simulink model "f14_digital"  (Simulink 7.6)
settings: Solver=ode45  SolverMode=SingleTasking  StartTime=0.0  StopTime=60  FixedStep=.01  RelTol=1e-4  AbsTol=1e-6
PreLoadFcn:
  | load f14_digital_data.mat
values from neighbouring files (symbols this model uses):
  a = 2.5348    [f14_digital_data.mat]    (also in f14dat_digital.m; sanim.m = size(vert); sanim3dof.m = size(vert))
  b = 64.13    [f14_digital_data.mat]    (also in f14dat_digital.m)
  deltat = pinput(23)    [aero_extkalman.m]    (also in aero_radplot.m = 1; f14_digital_data.mat = 0.1; f14dat_digital.m = 0.1)
  deltat1 = 0.01    [f14_digital_data.mat]    (also in f14dat_digital.m)
  fden = [1 188.495559215 17765.287922 837169.470368]    [f14_digital_data.mat]    (also in f14dat_digital.m = [ 1, 1.884955592153875e+02, 1.776528792196083e+04, 8.3716947)
  fnum = [0 0 0 837169.470368]    [f14_digital_data.mat]    (also in f14dat_digital.m = [ 0, 0, 0, 8.371694703680943e+05 ])
  g = 9.81    [aero_guid_dat.m]    (also in f14_digital_data.mat = 32.2; f14dat_digital.m = 32.2)
  Ka = 0.677    [f14_digital_data.mat]    (also in f14dat_digital.m)
  Kf = -1.746    [f14_digital_data.mat]    (also in f14dat_digital.m)
  Ki = -3.864    [f14_digital_data.mat]    (also in f14dat_digital.m)
  Kq = 0.8156    [f14_digital_data.mat]    (also in f14dat_digital.m)
  Md = -6.8847    [f14_digital_data.mat]    (also in f14dat_digital.m)
  Mq = -0.6571    [f14_digital_data.mat]    (also in f14dat_digital.m)
  Mw = -0.00592    [f14_digital_data.mat]    (also in f14dat_digital.m)
  Swg = 3    [f14_digital_data.mat]    (also in f14dat_digital.m)
  Tal = 0.3959    [f14_digital_data.mat]    (also in f14dat_digital.m)
  Ts = 0.1    [f14_digital_data.mat]    (also in f14dat_digital.m)
  Uo = 689.4    [f14_digital_data.mat]    (also in f14dat_digital.m)
  Vto = 690.4    [f14_digital_data.mat]    (also in f14dat_digital.m)
  W1 = 2.971    [f14_digital_data.mat]    (also in f14dat_digital.m)
  W2 = 4.144    [f14_digital_data.mat]    (also in f14dat_digital.m)
  Zd = -63.9979    [f14_digital_data.mat]    (also in f14dat_digital.m)
  Zw = -0.6385    [f14_digital_data.mat]    (also in f14dat_digital.m)
undefined symbols (not defined in the file or in its folder): DiscIntNeverNeededParam
libraries: simulink x5, f14actuator x1, cstblocks x1
Description:
  | High angle of attack mode for a digital flight control system
settings Model: Creator=The MathWorks Inc.  ExtModeTrigMode=oneshot  ExtModeArmWhenConnect=off  ExtModeAutoUpdateStatusClock=off
settings DataIOCC: ExternalInput=[]  InitialState=[]  LimitDataPoints=off  SaveOutput=off  SaveTime=off  SignalLoggingName=logsOut
settings OptimizationCC: BlockReduction=off  BooleanDataType=off  InlineInvariantSignals=on  InitFltsAndDblsToZero=on
settings DebuggingCC: SaveWithParameterizedLinksMsg=none  CheckExecutionContextPreStartOutputMsg=on  CheckExecutionContextRuntimeOutputMsg=on  SignalResolutionControl=TryResolveAllWithWarning  SolverPrmCheckMsg=none  MultiTaskDSMMsg=warning  MultiTaskCondExecSysMsg=none  SigSpecEnsureSampleTimeMsg=none  IntegerOverflowMsg=none
settings SFSimCC: SimParseCustomCode=off
settings RTWCC: GenCodeOnly=on  TemplateMakefile=grt_vc.tmf  IncludeERTFirstTime=on
settings CodeAppCC: CustomSymbolStrFcn=$F$N$M
settings GRTTargetCC: TargetFcnLib=ansi_tfl_tmw.mat

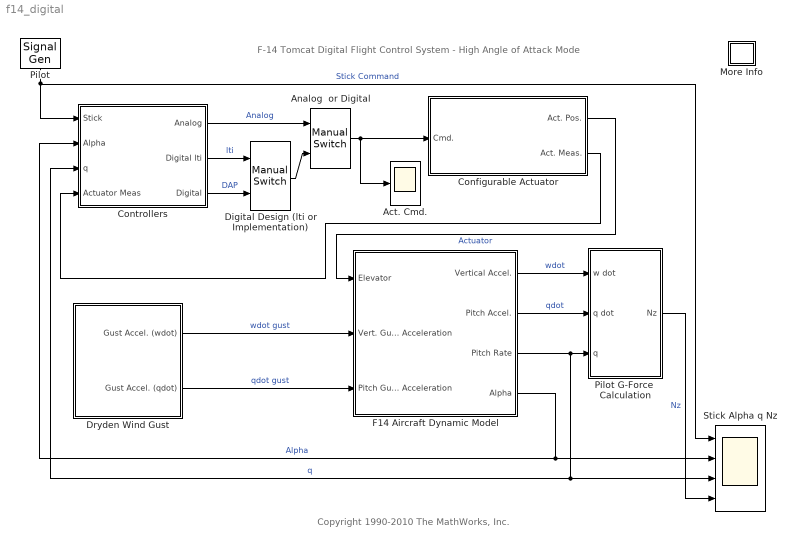
== system f14_digital ==
  note: Copyright 1990-2010 The MathWorks, Inc.
  note: F-14 Tomcat Digital Flight Control System - High Angle of Attack Mode
  Act. Cmd. : Scope
      settings: TickLabels=on  TimeRange=15  YMin=-2.5  YMax=2.5  DataFormat=Array
  Analog  or Digital : simulink/Signal Routing/Manual Switch  SystemSampleTime=-1  sw=1  action=0  varsize=off
  Configurable Actuator : Subsystem  BlockChoice=Linear Actuator Subsystem
      settings: MemberBlocks=Linear Actuator Subsystem,Non-Linear Actuator Subsystem
      settings: TemplateBlock=|
      | f14actuator/Configurable
      | Actuator
  Controllers : Subsystem
      mask Display: image(evalin('base','contrgb'))
  Digital Design (lti or Implementation) : simulink/Signal Routing/Manual Switch  SystemSampleTime=-1  sw=0  action=0  varsize=off
  Dryden Wind Gust : Subsystem
      mask Display: image(evalin('base','weatherrgb'))
  F14 Aircraft Dynamic Model : Subsystem
      mask Display: image(evalin('base','rgb'))
  More Info : Subsystem
      settings: OpenFcn=showdemo(bdroot(gcb))
      mask Display: disp('?')
  Pilot : SignalGenerator  WaveForm=square  Frequency=.1
  Pilot G-Force  Calculation : Subsystem
  Stick Alpha q Nz : Scope  NumInputPorts=4
      settings: TickLabels=on  TimeRange=15  YMin=-1~-1.5~-3~-15  YMax=1~1.5~3~15  DataFormat=Array
  wires:
  Controllers/3(Digital) -> Digital Design (lti or Implementation)/2  "DAP"
  Controllers/2(Digital lti) -> Digital Design (lti or Implementation)/1  "lti"
  Digital Design (lti or Implementation)/1 -> Analog  or Digital/2
  Configurable Actuator/1(Act. Pos.) -> F14 Aircraft Dynamic Model/1(Elevator)  "Actuator"
  Controllers/1(Analog) -> Analog  or Digital/1  "Analog"
  F14 Aircraft Dynamic Model/1(Vertical Accel.) -> Pilot G-Force  Calculation/1(w dot)  "wdot"
  F14 Aircraft Dynamic Model/2(Pitch Accel.) -> Pilot G-Force  Calculation/2(q dot)  "qdot"
  Pilot/1 -> Stick Alpha q Nz/1, Controllers/1(Stick)  "Stick Command"
  F14 Aircraft Dynamic Model/4(Alpha) -> Stick Alpha q Nz/2, Controllers/2(Alpha)  "Alpha"
  Configurable Actuator/2(Act. Meas.) -> Controllers/4(Actuator Meas)
  Dryden Wind Gust/2(Gust Accel. (qdot)) -> F14 Aircraft Dynamic Model/3(Pitch Gust Acceleration)  "qdot gust"
  Dryden Wind Gust/1(Gust Accel. (wdot)) -> F14 Aircraft Dynamic Model/2(Vert. Gust Acceleration)  "wdot gust"
  F14 Aircraft Dynamic Model/3(Pitch Rate) -> Pilot G-Force  Calculation/3(q), Stick Alpha q Nz/3, Controllers/3(q)  "q"
  Pilot G-Force  Calculation/1(Nz) -> Stick Alpha q Nz/4  "Nz"
  Analog  or Digital/1 -> Configurable Actuator/1(Cmd.), Act. Cmd./1

== system f14_digital/Configurable Actuator ==
  Cmd. : Inport
  Linear Actuator Subsystem : f14actuator/Linear Actuator Subsystem  SystemSampleTime=-1
  Act. Pos. : Outport
  Act. Meas. : Outport  Port=2
  wires:
  Cmd./1 -> Linear Actuator Subsystem/1
  Linear Actuator Subsystem/1 -> Act. Pos./1
  Linear Actuator Subsystem/2 -> Act. Meas./1

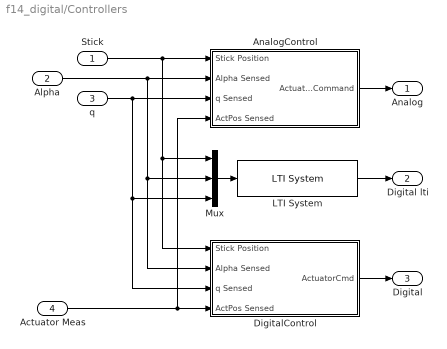
== system f14_digital/Controllers ==
  Stick : Inport
  Alpha : Inport  Port=2
  q : Inport  Port=3
  Actuator Meas : Inport  Port=4
  AnalogControl : Subsystem
  DigitalControl : Subsystem
  LTI System : cstblocks/LTI System  sys=discap  IC=[0]
  Mux : Mux  Inputs=3
  Analog : Outport
  Digital lti : Outport  Port=2
  Digital : Outport  Port=3
  wires:
  Stick/1 -> AnalogControl/1(Stick Position), DigitalControl/1(Stick Position), Mux/1
  Actuator Meas/1 -> DigitalControl/4(ActPos Sensed), AnalogControl/4(ActPos Sensed)
  LTI System/1 -> Digital lti/1
  DigitalControl/1(ActuatorCmd) -> Digital/1
  AnalogControl/1(Actuator Command) -> Analog/1
  Mux/1 -> LTI System/1
  Alpha/1 -> AnalogControl/2(Alpha Sensed), DigitalControl/2(Alpha Sensed), Mux/2
  q/1 -> AnalogControl/3(q Sensed), DigitalControl/3(q Sensed), Mux/3

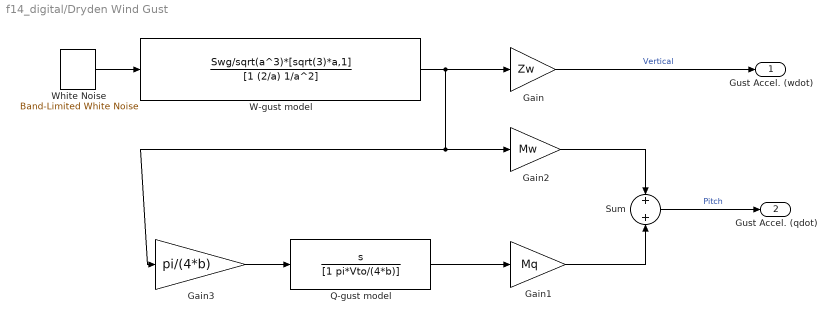
== system f14_digital/Dryden Wind Gust ==
  Gain : Gain  Gain=Zw  SaturateOnIntegerOverflow=on  OutDataTypeStr=Inherit: Same as input  ParamDataTypeStr=Inherit: Same as input
  Gain1 : Gain  Gain=Mq  SaturateOnIntegerOverflow=on  OutDataTypeStr=Inherit: Same as input  ParamDataTypeStr=Inherit: Same as input
  Gain2 : Gain  Gain=Mw  SaturateOnIntegerOverflow=on  OutDataTypeStr=Inherit: Same as input  ParamDataTypeStr=Inherit: Same as input
  Gain3 : Gain  Gain=pi/(4*b)  SaturateOnIntegerOverflow=on  OutDataTypeStr=Inherit: Same as input  ParamDataTypeStr=Inherit: Same as input
  Q-gust model : TransferFcn  Numerator=[1 0]  Denominator=[1 pi*Vto/(4*b)]
  Sum : Sum  SaturateOnIntegerOverflow=on  InputSameDT=on  OutDataTypeStr=Inherit: Same as first input
  W-gust model : TransferFcn  Numerator=Swg/sqrt(a^3)*[sqrt(3)*a,1]  Denominator=[1 (2/a) 1/a^2]
  White Noise : simulink/Sources/Band-Limited White Noise  Cov=10  Ts=0.01  seed=23341
  Gust Accel. (wdot) : Outport
  Gust Accel. (qdot) : Outport  Port=2
  wires:
  Gain/1 -> Gust Accel. (wdot)/1  "Vertical"
  White Noise/1 -> W-gust model/1
  Gain3/1 -> Q-gust model/1
  Sum/1 -> Gust Accel. (qdot)/1  "Pitch"
  Gain2/1 -> Sum/1
  Gain1/1 -> Sum/2
  Q-gust model/1 -> Gain1/1
  W-gust model/1 -> Gain/1, Gain2/1, Gain3/1

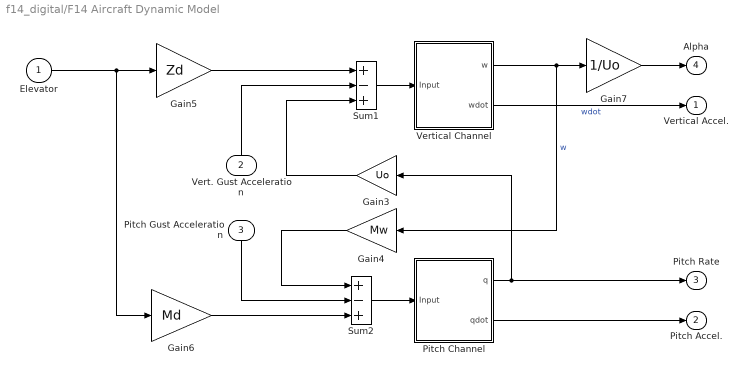
== system f14_digital/F14 Aircraft Dynamic Model ==
  Elevator : Inport
  Vert. Gust Acceleration : Inport  Port=2
  Pitch Gust Acceleration : Inport  Port=3
  Gain3 : Gain  Gain=Uo  SaturateOnIntegerOverflow=on  OutDataTypeStr=Inherit: Same as input  ParamDataTypeStr=Inherit: Same as input
  Gain4 : Gain  Gain=Mw  SaturateOnIntegerOverflow=on  OutDataTypeStr=Inherit: Same as input  ParamDataTypeStr=Inherit: Same as input
  Gain5 : Gain  Gain=Zd  SaturateOnIntegerOverflow=on  OutDataTypeStr=Inherit: Same as input  ParamDataTypeStr=Inherit: Same as input
  Gain6 : Gain  Gain=Md  SaturateOnIntegerOverflow=on  OutDataTypeStr=Inherit: Same as input  ParamDataTypeStr=Inherit: Same as input
  Gain7 : Gain  Gain=1/Uo  SaturateOnIntegerOverflow=on  OutDataTypeStr=Inherit: Same as input  ParamDataTypeStr=Inherit: Same as input
  Pitch Channel : Subsystem
  Sum1 : Sum  Inputs=+-+  SaturateOnIntegerOverflow=on  InputSameDT=on  OutDataTypeStr=Inherit: Same as first input
  Sum2 : Sum  Inputs=+-+  SaturateOnIntegerOverflow=on  InputSameDT=on  OutDataTypeStr=Inherit: Same as first input
  Vertical Channel : Subsystem
  Vertical Accel. : Outport
  Pitch Accel. : Outport  Port=2
  Pitch Rate : Outport  Port=3
  Alpha : Outport  Port=4
  wires:
  Pitch Channel/2(qdot) -> Pitch Accel./1
  Pitch Channel/1(q) -> Pitch Rate/1, Gain3/1
  Vertical Channel/2(wdot) -> Vertical Accel./1  "wdot"
  Vertical Channel/1(w) -> Gain4/1, Gain7/1  "w"
  Sum1/1 -> Vertical Channel/1(Input)
  Gain6/1 -> Sum2/3
  Gain5/1 -> Sum1/1
  Pitch Gust Acceleration/1 -> Sum2/2
  Sum2/1 -> Pitch Channel/1(Input)
  Vert. Gust Acceleration/1 -> Sum1/2
  Elevator/1 -> Gain5/1, Gain6/1
  Gain7/1 -> Alpha/1
  Gain3/1 -> Sum1/3
  Gain4/1 -> Sum2/1

== system f14_digital/More Info ==

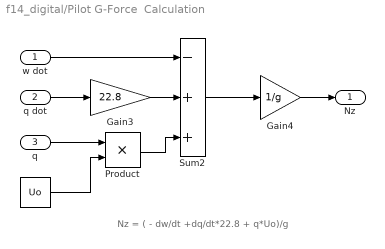
== system f14_digital/Pilot G-Force  Calculation ==
  note: Nz = ( - dw/dt +dq/dt*22.8 + q*Uo)/g
  w dot : Inport
  q dot : Inport  Port=2
  q : Inport  Port=3
  " " : Constant  Value=Uo
  Gain3 : Gain  Gain=22.8  SaturateOnIntegerOverflow=on  OutDataTypeStr=Inherit: Same as input  ParamDataTypeStr=Inherit: Same as input
  Gain4 : Gain  Gain=1/g  SaturateOnIntegerOverflow=on  OutDataTypeStr=Inherit: Same as input  ParamDataTypeStr=Inherit: Same as input
  Product : Product  SaturateOnIntegerOverflow=on  RndMeth=Zero  InputSameDT=on  OutDataTypeStr=Inherit: Same as first input
  Sum2 : Sum  Inputs=-++  SaturateOnIntegerOverflow=on  InputSameDT=on  OutDataTypeStr=Inherit: Same as first input
  Nz : Outport
  wires:
  Sum2/1 -> Gain4/1
  w dot/1 -> Sum2/1
  Gain4/1 -> Nz/1
  q dot/1 -> Gain3/1
  Gain3/1 -> Sum2/2
  Product/1 -> Sum2/3
  q/1 -> Product/1
  " "/1 -> Product/2

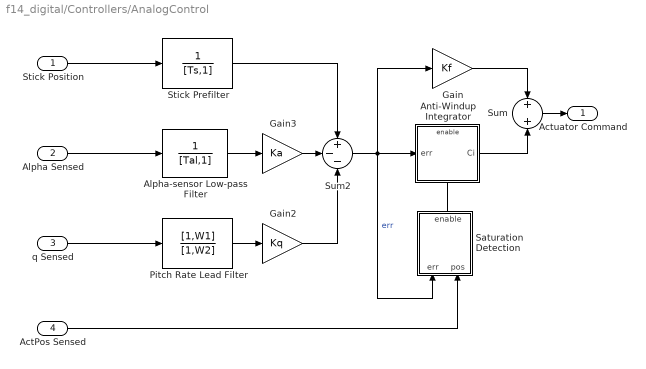
== system f14_digital/Controllers/AnalogControl ==
  Stick Position : Inport
  Alpha Sensed : Inport  Port=2
  q Sensed : Inport  Port=3
  ActPos Sensed : Inport  Port=4
  Alpha-sensor Low-pass Filter : TransferFcn  Denominator=[Tal,1]
  Anti-Windup Integrator : Subsystem  TreatAsAtomicUnit=on
      settings: RTWSystemCode=Inline
  Gain : Gain  Gain=Kf  SaturateOnIntegerOverflow=on  OutDataTypeStr=Inherit: Same as input  ParamDataTypeStr=Inherit: Same as input
  Gain2 : Gain  Gain=Kq  SaturateOnIntegerOverflow=on  OutDataTypeStr=Inherit: Same as input  ParamDataTypeStr=Inherit: Same as input
  Gain3 : Gain  Gain=Ka  SaturateOnIntegerOverflow=on  OutDataTypeStr=Inherit: Same as input  ParamDataTypeStr=Inherit: Same as input
  Pitch Rate Lead Filter : TransferFcn  Numerator=[1,W1]  Denominator=[1,W2]
  Saturation Detection : Subsystem
  Stick Prefilter : TransferFcn  Denominator=[Ts,1]
  Sum : Sum  Inputs=2  SaturateOnIntegerOverflow=on  InputSameDT=on  OutDataTypeStr=Inherit: Same as first input
  Sum2 : Sum  Inputs=+--  SaturateOnIntegerOverflow=on  InputSameDT=on  OutDataTypeStr=Inherit: Same as first input
  Actuator Command : Outport
  wires:
  Sum2/1 -> Gain/1, Anti-Windup Integrator/1(err), Saturation Detection/1(err)  "err"
  Anti-Windup Integrator/1(Ci) -> Sum/2
  Sum/1 -> Actuator Command/1
  Stick Position/1 -> Stick Prefilter/1
  Alpha-sensor Low-pass Filter/1 -> Gain3/1
  Gain2/1 -> Sum2/3
  Stick Prefilter/1 -> Sum2/1
  Pitch Rate Lead Filter/1 -> Gain2/1
  Gain3/1 -> Sum2/2
  Gain/1 -> Sum/1
  Alpha Sensed/1 -> Alpha-sensor Low-pass Filter/1
  q Sensed/1 -> Pitch Rate Lead Filter/1
  ActPos Sensed/1 -> Saturation Detection/2(pos)
  Saturation Detection/1(enable) -> Anti-Windup Integrator/Enable

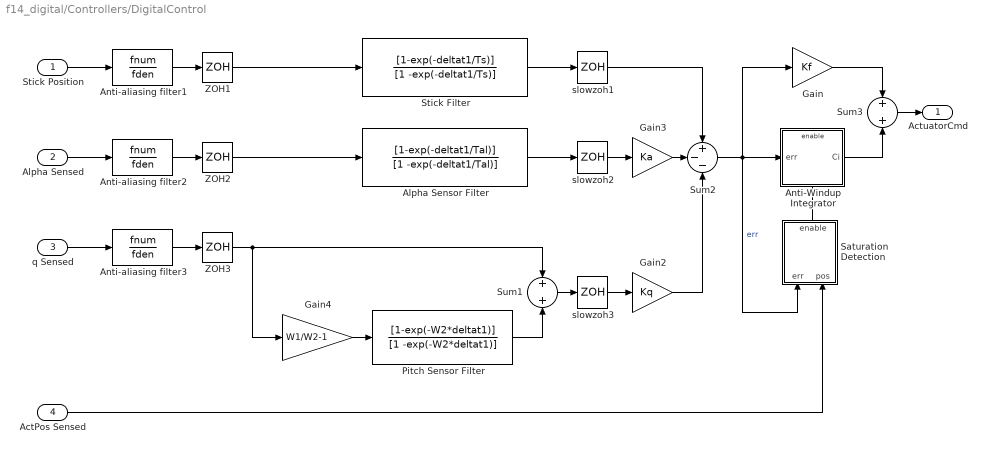
== system f14_digital/Controllers/DigitalControl ==
  Stick Position : Inport
  Alpha Sensed : Inport  Port=2
  q Sensed : Inport  Port=3
  ActPos Sensed : Inport  Port=4
  Alpha Sensor Filter : DiscreteTransferFcn  Numerator=[1-exp(-deltat1/Tal)]  Denominator=[1 -exp(-deltat1/Tal)]  SampleTime=deltat1
  Anti-Windup Integrator : Subsystem  TreatAsAtomicUnit=on
      settings: RTWSystemCode=Inline
  Anti-aliasing filter1 : TransferFcn  Numerator=fnum  Denominator=fden
      settings: AttributesFormatString=%<Description>
  Anti-aliasing filter2 : TransferFcn  Numerator=fnum  Denominator=fden
      settings: AttributesFormatString=%<Description>
  Anti-aliasing filter3 : TransferFcn  Numerator=fnum  Denominator=fden
      settings: AttributesFormatString=%<Description>
  Gain : Gain  Gain=Kf  SaturateOnIntegerOverflow=on  OutDataTypeStr=Inherit: Same as input  ParamDataTypeStr=Inherit: Same as input
  Gain2 : Gain  Gain=Kq  SaturateOnIntegerOverflow=on  OutDataTypeStr=Inherit: Same as input  ParamDataTypeStr=Inherit: Same as input
  Gain3 : Gain  Gain=Ka  SaturateOnIntegerOverflow=on  OutDataTypeStr=Inherit: Same as input  ParamDataTypeStr=Inherit: Same as input
  Gain4 : Gain  Gain=W1/W2-1  SaturateOnIntegerOverflow=on  OutDataTypeStr=Inherit: Same as input  ParamDataTypeStr=Inherit: Same as input
  Pitch Sensor Filter : DiscreteTransferFcn  Numerator=[1-exp(-W2*deltat1)]  Denominator=[1 -exp(-W2*deltat1)]  SampleTime=deltat1
  Saturation Detection : Subsystem
  Stick Filter : DiscreteTransferFcn  Numerator=[1-exp(-deltat1/Ts)]  Denominator=[1 -exp(-deltat1/Ts)]  SampleTime=deltat1
  Sum1 : Sum  Inputs=2  SaturateOnIntegerOverflow=on  InputSameDT=on  OutDataTypeStr=Inherit: Same as first input
  Sum2 : Sum  Inputs=+--  SaturateOnIntegerOverflow=on  InputSameDT=on  OutDataTypeStr=Inherit: Same as first input
  Sum3 : Sum  Inputs=2  SaturateOnIntegerOverflow=on  InputSameDT=on  OutDataTypeStr=Inherit: Same as first input
  ZOH1 : ZeroOrderHold  SampleTime=deltat1
  ZOH2 : ZeroOrderHold  SampleTime=deltat1
  ZOH3 : ZeroOrderHold  SampleTime=deltat1
  slowzoh1 : ZeroOrderHold  SampleTime=deltat
  slowzoh2 : ZeroOrderHold  SampleTime=deltat
  slowzoh3 : ZeroOrderHold  SampleTime=deltat
  ActuatorCmd : Outport
  wires:
  Sum3/1 -> ActuatorCmd/1
  Sum2/1 -> Gain/1, Anti-Windup Integrator/1(err), Saturation Detection/1(err)  "err"
  Alpha Sensed/1 -> Anti-aliasing filter2/1
  Stick Filter/1 -> slowzoh1/1
  slowzoh1/1 -> Sum2/1
  Alpha Sensor Filter/1 -> slowzoh2/1
  slowzoh2/1 -> Gain3/1
  Gain3/1 -> Sum2/2
  Gain/1 -> Sum3/1
  Anti-Windup Integrator/1(Ci) -> Sum3/2
  Gain2/1 -> Sum2/3
  q Sensed/1 -> Anti-aliasing filter3/1
  Sum1/1 -> slowzoh3/1
  Pitch Sensor Filter/1 -> Sum1/2
  Gain4/1 -> Pitch Sensor Filter/1
  slowzoh3/1 -> Gain2/1
  Stick Position/1 -> Anti-aliasing filter1/1
  ZOH1/1 -> Stick Filter/1
  Anti-aliasing filter1/1 -> ZOH1/1
  Anti-aliasing filter2/1 -> ZOH2/1
  Anti-aliasing filter3/1 -> ZOH3/1
  ZOH2/1 -> Alpha Sensor Filter/1
  ZOH3/1 -> Sum1/1, Gain4/1
  Saturation Detection/1(enable) -> Anti-Windup Integrator/Enable
  ActPos Sensed/1 -> Saturation Detection/2(pos)

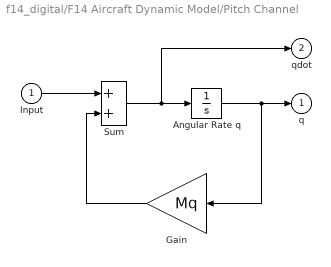
== system f14_digital/F14 Aircraft Dynamic Model/Pitch Channel ==
  Input : Inport
  "Angular Rate q " : Integrator
  Gain : Gain  Gain=Mq  SaturateOnIntegerOverflow=on  OutDataTypeStr=Inherit: Same as input  ParamDataTypeStr=Inherit: Same as input
  Sum : Sum  SaturateOnIntegerOverflow=on  InputSameDT=on  OutDataTypeStr=Inherit: Same as first input
  q : Outport
  qdot : Outport  Port=2
  wires:
  Input/1 -> Sum/1
  Gain/1 -> Sum/2
  "Angular Rate q "/1 -> q/1, Gain/1
  Sum/1 -> "Angular Rate q "/1, qdot/1

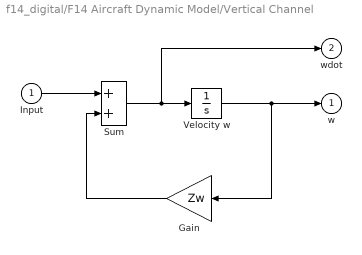
== system f14_digital/F14 Aircraft Dynamic Model/Vertical Channel ==
  Input : Inport
  Gain : Gain  Gain=Zw  SaturateOnIntegerOverflow=on  OutDataTypeStr=Inherit: Same as input  ParamDataTypeStr=Inherit: Same as input
  Sum : Sum  SaturateOnIntegerOverflow=on  InputSameDT=on  OutDataTypeStr=Inherit: Same as first input
  Velocity w : Integrator
  w : Outport
  wdot : Outport  Port=2
  wires:
  Sum/1 -> wdot/1, Velocity w/1
  Velocity w/1 -> Gain/1, w/1
  Gain/1 -> Sum/2
  Input/1 -> Sum/1

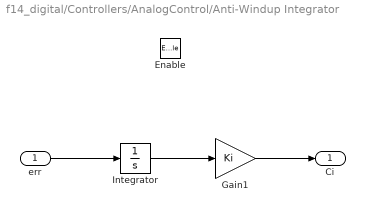
== system f14_digital/Controllers/AnalogControl/Anti-Windup Integrator ==
  err : Inport
  Enable : EnablePort
  Gain1 : Gain  Gain=Ki  SaturateOnIntegerOverflow=on  OutDataTypeStr=Inherit: Same as input  ParamDataTypeStr=Inherit: Same as input
  Integrator : Integrator
  Ci : Outport  InitialOutput=0
  wires:
  err/1 -> Integrator/1
  Integrator/1 -> Gain1/1
  Gain1/1 -> Ci/1

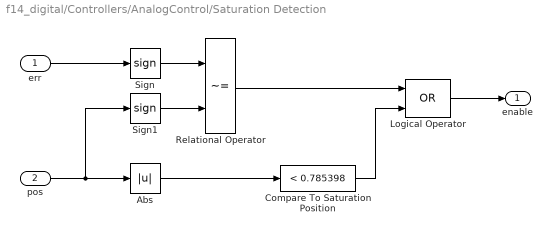
== system f14_digital/Controllers/AnalogControl/Saturation Detection ==
  err : Inport
  pos : Inport  Port=2
  Abs : Abs  ZeroCross=off
  Compare To Saturation Position : simulink/Logic and Bit Operations/Compare To Constant  relop=<  const=0.785398  LogicOutDataTypeMode=boolean  ZeroCross=off
  Logical Operator : Logic  Operator=OR  AllPortsSameDT=off  OutDataTypeStr=boolean
  Relational Operator : RelationalOperator  Operator=~=  OutDataTypeStr=boolean  ZeroCross=off
  Sign : Signum  ZeroCross=off
  Sign1 : Signum  ZeroCross=off
  enable : Outport
  wires:
  pos/1 -> Sign1/1, Abs/1
  Sign/1 -> Relational Operator/1
  Relational Operator/1 -> Logical Operator/1
  Compare To Saturation Position/1 -> Logical Operator/2
  Sign1/1 -> Relational Operator/2
  Abs/1 -> Compare To Saturation Position/1
  err/1 -> Sign/1
  Logical Operator/1 -> enable/1

== system f14_digital/Controllers/DigitalControl/Anti-Windup Integrator ==
  err : Inport
  Enable : EnablePort
  Discrete-Time Integrator : DiscreteIntegrator  IntegratorMethod=Integration: Trapezoidal  SampleTime=deltat  ICPrevOutput=DiscIntNeverNeededParam  ICPrevScaledInput=DiscIntNeverNeededParam
  Gain1 : Gain  Gain=Ki  SaturateOnIntegerOverflow=on  OutDataTypeStr=Inherit: Same as input  ParamDataTypeStr=Inherit: Same as input
  Ci : Outport  InitialOutput=0
  wires:
  err/1 -> Discrete-Time Integrator/1
  Discrete-Time Integrator/1 -> Gain1/1
  Gain1/1 -> Ci/1

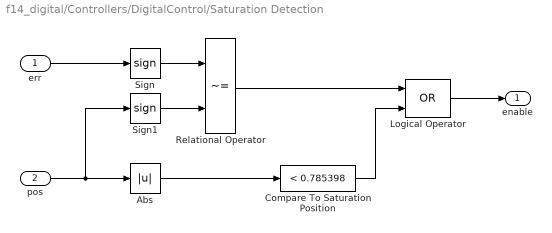
== system f14_digital/Controllers/DigitalControl/Saturation Detection ==
  err : Inport
  pos : Inport  Port=2
  Abs : Abs  ZeroCross=off
  Compare To Saturation Position : simulink/Logic and Bit Operations/Compare To Constant  relop=<  const=0.785398  LogicOutDataTypeMode=boolean  ZeroCross=off
  Logical Operator : Logic  Operator=OR  AllPortsSameDT=off  OutDataTypeStr=boolean
  Relational Operator : RelationalOperator  Operator=~=  OutDataTypeStr=boolean  ZeroCross=off
  Sign : Signum  ZeroCross=off
  Sign1 : Signum  ZeroCross=off
  enable : Outport
  wires:
  pos/1 -> Sign1/1, Abs/1
  Sign/1 -> Relational Operator/1
  Relational Operator/1 -> Logical Operator/1
  Compare To Saturation Position/1 -> Logical Operator/2
  Sign1/1 -> Relational Operator/2
  Abs/1 -> Compare To Saturation Position/1
  err/1 -> Sign/1
  Logical Operator/1 -> enable/1
